simulink model "BMTM8_vExp2_prot2"  (R2018b)
settings: Solver=FixedStepAuto  StartTime=0.0  StopTime=max(phi_laser_space(:,1))  FixedStep=1e-3  RelTol=1e-3
settings Model: Creator=BuitenwegJR  LastModifiedBy=BuitenwegJR

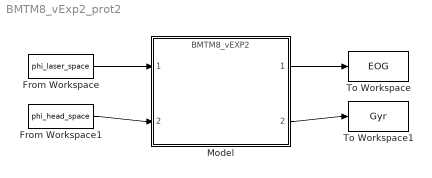
== system BMTM8_vExp2_prot2 ==
  From Workspace : FromWorkspace  VariableName=phi_laser_space  SampleTime=0
  From Workspace1 : FromWorkspace  VariableName=phi_head_space  SampleTime=0
  Model : ModelReference  ModelNameDialog=BMTM8_vEXP2.slxp  ModelReferenceVersion=1.7  CopyOfModelProtected=on
  To Workspace : ToWorkspace  VariableName=EOG  SaveFormat=Timeseries  SampleTime=-1
  To Workspace1 : ToWorkspace  VariableName=Gyr  SaveFormat=Timeseries  SampleTime=-1
  wires:
  From Workspace/1 -> Model/1
  From Workspace1/1 -> Model/2
  Model/1 -> To Workspace/1
  Model/2 -> To Workspace1/1
